simulink model "Seccion_h2022"  (R2022a)
settings: Solver=VariableStepAuto  StartTime=0.0  StopTime=12  RelTol=1e-3
undefined symbols (not defined in the file): C_L
settings Model: Creator=Admin  LastModifiedBy=gonza

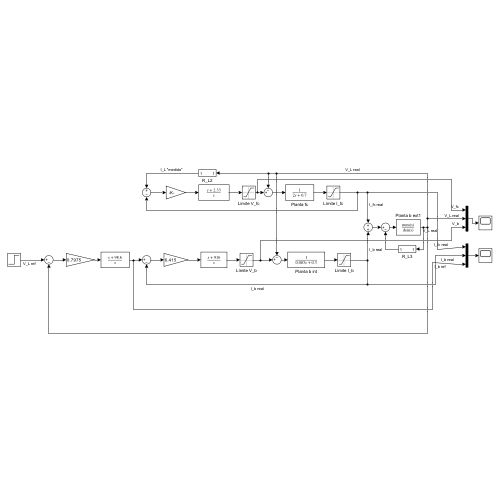
[thumbnail: Simulink's stored preview of the top-level diagram]
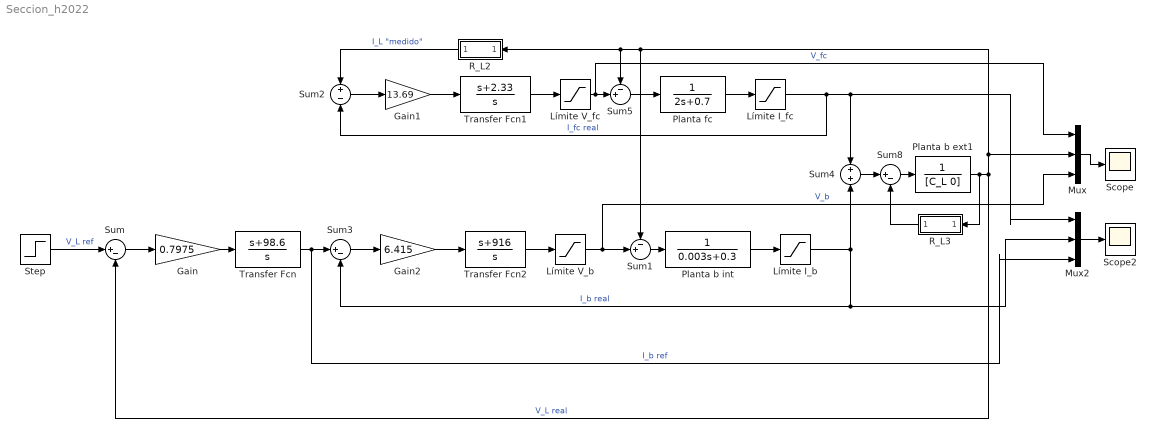
== system Seccion_h2022 ==
  Gain : Gain  Gain=0.7975
  Gain1 : Gain  Gain=13.69
  Gain2 : Gain  Gain=6.415
  Límite I_b : Saturate  UpperLimit=120  LowerLimit=-120
  Límite I_fc : Saturate  UpperLimit=200  LowerLimit=0
  Límite V_b : Saturate  UpperLimit=400  LowerLimit=-400
  Límite V_fc : Saturate  UpperLimit=450  LowerLimit=0
  Mux : Mux  Inputs=3
  Mux2 : Mux  Inputs=3
  Planta b ext1 : TransferFcn  Numerator=1  Denominator=[C_L 0]
  Planta b int : TransferFcn  Denominator=[0.003 0.3]
  Planta fc : TransferFcn  Denominator=[2 0.7]
  R_L2 : Subsystem
  R_L3 : Subsystem
  Scope : Scope
  Scope2 : Scope
  Step : Step  Time=0.1  After=250  SampleTime=0
  Sum : Sum  Inputs=|+-
  Sum1 : Sum  Inputs=-+|
  Sum2 : Sum  Inputs=+|-
  Sum3 : Sum  Inputs=|+-
  Sum4 : Sum  Inputs=+|+
  Sum5 : Sum  Inputs=-+|
  Sum8 : Sum  Inputs=|+-
  Transfer Fcn : TransferFcn  Numerator=[1 98.6]  Denominator=[1 0]
  Transfer Fcn1 : TransferFcn  Numerator=[1 2.33]  Denominator=[1 0]
  Transfer Fcn2 : TransferFcn  Numerator=[1 916]  Denominator=[1 0]
  wires:
  Step/1 -> Sum/1  "V_L ref"
  Sum/1 -> Gain/1
  Gain/1 -> Transfer Fcn/1
  Transfer Fcn/1 -> Mux2/3, Sum3/1  "I_b ref"
  Gain1/1 -> Transfer Fcn1/1
  Sum2/1 -> Gain1/1
  Sum3/1 -> Gain2/1
  Gain2/1 -> Transfer Fcn2/1
  Transfer Fcn1/1 -> Límite V_fc/1
  Transfer Fcn2/1 -> Límite V_b/1
  Sum4/1 -> Sum8/1
  Planta b ext1/1 -> R_L3/1(In1), R_L2/1(In1), Sum5/1, Sum1/1, Mux/2, Sum/2  "V_L real"
  Mux/1 -> Scope/1
  Límite I_b/1 -> Sum3/2, Mux2/2, Sum4/2  "I_b real"
  Límite I_fc/1 -> Sum2/2, Sum4/1, Mux2/1  "I_fc real"
  Planta b int/1 -> Límite I_b/1
  Planta fc/1 -> Límite I_fc/1
  R_L2/1(Out1) -> Sum2/1  "I_L \"medido\""
  Límite V_b/1 -> Mux/3, Sum1/2  "V_b"
  Sum1/1 -> Planta b int/1
  Límite V_fc/1 -> Mux/1, Sum5/2  "V_fc"
  Sum5/1 -> Planta fc/1
  Mux2/1 -> Scope2/1
  Sum8/1 -> Planta b ext1/1
  R_L3/1(Out1) -> Sum8/2

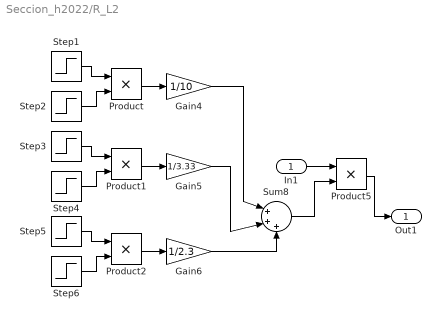
== system Seccion_h2022/R_L2 ==
  In1 : Inport
  Gain4 : Gain  Gain=1/10
  Gain5 : Gain  Gain=1/3.33
  Gain6 : Gain  Gain=1/2.3
  Product{,1..2,5} (4 alike) : Product
  Step1 : Step  Time=0.1  SampleTime=0
  Step2 : Step  Time=2.1  Before=1  After=0  SampleTime=0
  Step3 : Step  Time=2.1  SampleTime=0
  Step4 : Step  Time=5.1  Before=1  After=0  SampleTime=0
  Step5 : Step  Time=5.1  SampleTime=0
  Step6 : Step  Time=8.1  Before=1  After=0  SampleTime=0
  Sum8 : Sum  Inputs=|+++
  Out1 : Outport
  wires:
  Step2/1 -> Product/2
  Step3/1 -> Product1/1
  Product/1 -> Gain4/1
  Step4/1 -> Product1/2
  Product1/1 -> Gain5/1
  Gain4/1 -> Sum8/1
  Step6/1 -> Product2/2
  Step5/1 -> Product2/1
  Product2/1 -> Gain6/1
  Step1/1 -> Product/1
  Gain5/1 -> Sum8/2
  Gain6/1 -> Sum8/3
  Product5/1 -> Out1/1
  In1/1 -> Product5/1
  Sum8/1 -> Product5/2

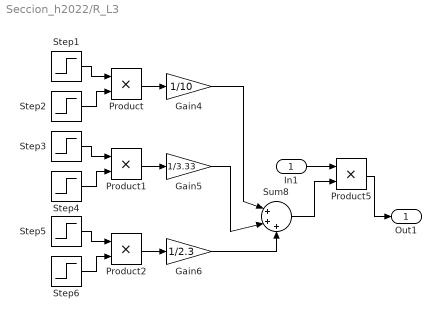
== system Seccion_h2022/R_L3 ==
  In1 : Inport
  Gain4 : Gain  Gain=1/10
  Gain5 : Gain  Gain=1/3.33
  Gain6 : Gain  Gain=1/2.3
  Product{,1..2,5} (4 alike) : Product
  Step1 : Step  Time=0.1  SampleTime=0
  Step2 : Step  Time=2.1  Before=1  After=0  SampleTime=0
  Step3 : Step  Time=2.1  SampleTime=0
  Step4 : Step  Time=5.1  Before=1  After=0  SampleTime=0
  Step5 : Step  Time=5.1  SampleTime=0
  Step6 : Step  Time=8.1  Before=1  After=0  SampleTime=0
  Sum8 : Sum  Inputs=|+++
  Out1 : Outport
  wires:
  Step2/1 -> Product/2
  Step3/1 -> Product1/1
  Product/1 -> Gain4/1
  Step4/1 -> Product1/2
  Product1/1 -> Gain5/1
  Gain4/1 -> Sum8/1
  Step6/1 -> Product2/2
  Step5/1 -> Product2/1
  Product2/1 -> Gain6/1
  Step1/1 -> Product/1
  Gain5/1 -> Sum8/2
  Gain6/1 -> Sum8/3
  Product5/1 -> Out1/1
  In1/1 -> Product5/1
  Sum8/1 -> Product5/2
